simulink model "tests_inverse_shapers"  (R2015b)
settings: Solver=VariableStepAuto  StartTime=0.0  StopTime=10.0  RelTol=1e-3
undefined symbols (not defined in the file): a, alpha, tau
libraries: cstblocks x1
settings Model: Creator=dave  LastModifiedBy=dave

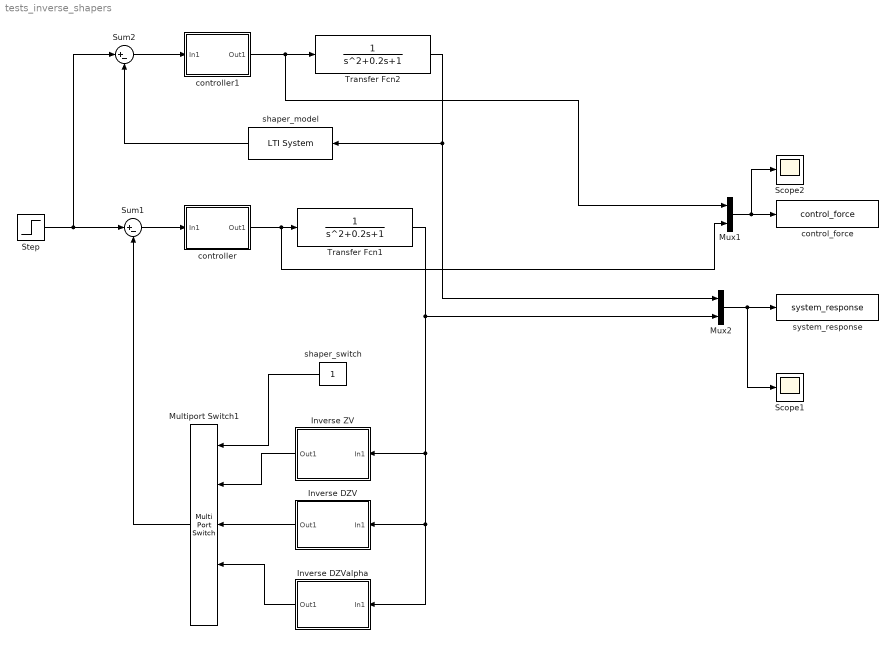
== system tests_inverse_shapers ==
  Inverse DZV : Subsystem
  Inverse DZValpha : Subsystem
  Inverse ZV : Subsystem
  Multiport Switch1 : MultiPortSwitch  Inputs=4
  Mux1 : Mux  Inputs=2
  Mux2 : Mux  Inputs=2
  Scope1 : Scope
  Scope2 : Scope
  Step : Step  SampleTime=0
  Sum1 : Sum  Inputs=|+-
  Sum2 : Sum  Inputs=|+-
  Transfer Fcn1 : TransferFcn  Denominator=[1 0.2 1]
  Transfer Fcn2 : TransferFcn  Denominator=[1 0.2 1]
  control_force : ToWorkspace  VariableName=control_force  SaveFormat=Timeseries  SampleTime=-1
  controller : Subsystem
  controller1 : Subsystem
  shaper_model : cstblocks/LTI System  sys=shaper_model  IC=[]
  shaper_switch : Constant
  system_response : ToWorkspace  VariableName=system_response  SaveFormat=Timeseries  SampleTime=-1
  wires:
  Step/1 -> Sum2/1, Sum1/1
  Sum1/1 -> controller/1(In1)
  controller/1(Out1) -> Mux1/2, Transfer Fcn1/1
  Sum2/1 -> controller1/1(In1)
  controller1/1(Out1) -> Mux1/1, Transfer Fcn2/1
  shaper_model/1 -> Sum2/2
  Mux2/1 -> Scope1/1, system_response/1
  Transfer Fcn2/1 -> Mux2/1, shaper_model/1
  Transfer Fcn1/1 -> Inverse DZValpha/1(In1), Inverse DZV/1(In1), Inverse ZV/1(In1), Mux2/2
  Mux1/1 -> Scope2/1, control_force/1
  Inverse DZValpha/1(Out1) -> Multiport Switch1/4
  Inverse DZV/1(Out1) -> Multiport Switch1/3
  Inverse ZV/1(Out1) -> Multiport Switch1/2
  shaper_switch/1 -> Multiport Switch1/1
  Multiport Switch1/1 -> Sum1/2

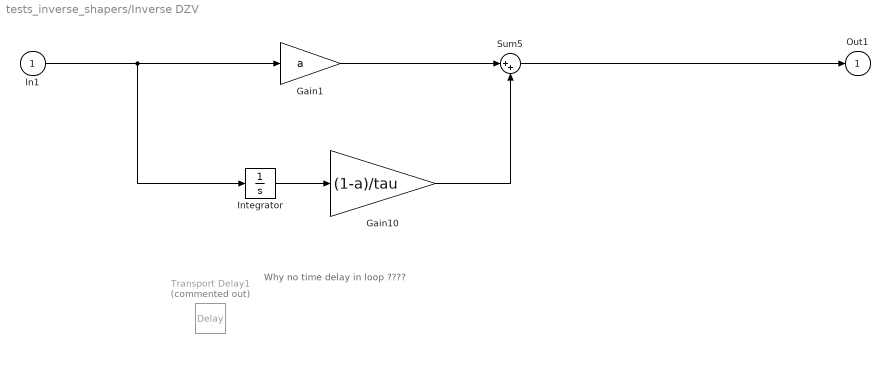
== system tests_inverse_shapers/Inverse DZV ==
  note: Why no time delay in loop ????
  In1 : Inport
  Gain1 : Gain  Gain=a
  Gain10 : Gain  Gain=(1-a)/tau
  Integrator : Integrator  LimitOutput=on  UpperSaturationLimit=tau  LowerSaturationLimit=0
  Sum5 : Sum  Inputs=|++
  Transport Delay1 : TransportDelay  Commented=on  DelayTime=tau
  Out1 : Outport
  wires:
  Sum5/1 -> Out1/1
  Integrator/1 -> Gain10/1
  Gain10/1 -> Sum5/2
  Gain1/1 -> Sum5/1
  In1/1 -> Integrator/1, Gain1/1

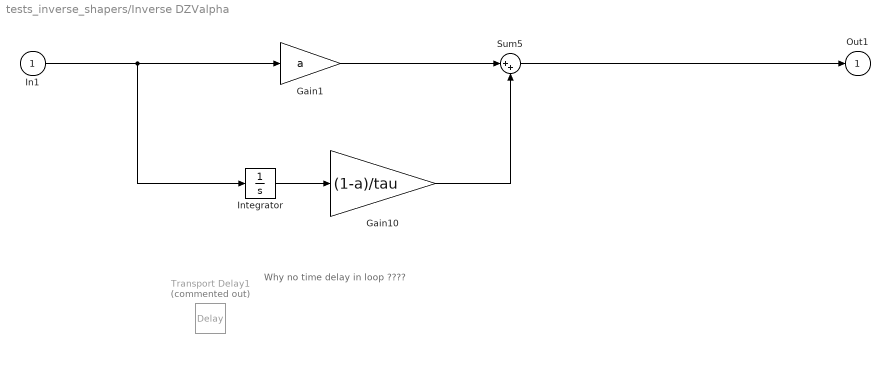
== system tests_inverse_shapers/Inverse DZValpha ==
  note: Why no time delay in loop ????
  In1 : Inport
  Gain1 : Gain  Gain=a
  Gain10 : Gain  Gain=(1-a)/tau
  Integrator : Integrator  LimitOutput=on  UpperSaturationLimit=tau  LowerSaturationLimit=0
  Sum5 : Sum  Inputs=|++
  Transport Delay1 : TransportDelay  Commented=on  DelayTime=tau
  Out1 : Outport
  wires:
  In1/1 -> Gain1/1, Integrator/1
  Gain1/1 -> Sum5/1
  Gain10/1 -> Sum5/2
  Integrator/1 -> Gain10/1
  Sum5/1 -> Out1/1

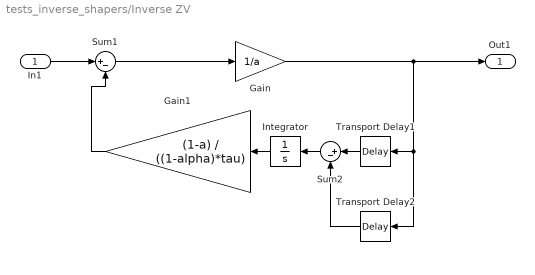
== system tests_inverse_shapers/Inverse ZV ==
  In1 : Inport
  Gain : Gain  Gain=1/a
  Gain1 : Gain  Gain=(1-a) / ((1-alpha)*tau)
  Integrator : Integrator  LimitOutput=on  UpperSaturationLimit=tau  LowerSaturationLimit=0
  Sum1 : Sum  Inputs=|+-
  Sum2 : Sum  Inputs=|+-
  Transport Delay1 : TransportDelay  DelayTime=tau*alpha
  Transport Delay2 : TransportDelay  DelayTime=tau
  Out1 : Outport
  wires:
  Gain/1 -> Transport Delay2/1, Transport Delay1/1, Out1/1
  Gain1/1 -> Sum1/2
  Sum1/1 -> Gain/1
  In1/1 -> Sum1/1
  Integrator/1 -> Gain1/1
  Transport Delay2/1 -> Sum2/2
  Sum2/1 -> Integrator/1
  Transport Delay1/1 -> Sum2/1

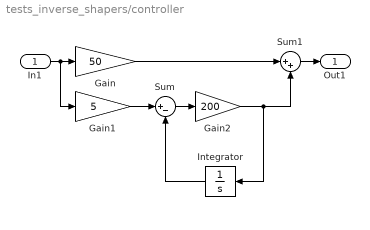
== system tests_inverse_shapers/controller ==
  In1 : Inport
  Gain : Gain  Gain=50
  Gain1 : Gain  Gain=5
  Gain2 : Gain  Gain=200
  Integrator : Integrator
  Sum : Sum  Inputs=|+-
  Sum1 : Sum  Inputs=|++
  Out1 : Outport
  wires:
  Gain/1 -> Sum1/1
  Gain1/1 -> Sum/1
  In1/1 -> Gain1/1, Gain/1
  Sum/1 -> Gain2/1
  Gain2/1 -> Sum1/2, Integrator/1
  Integrator/1 -> Sum/2
  Sum1/1 -> Out1/1

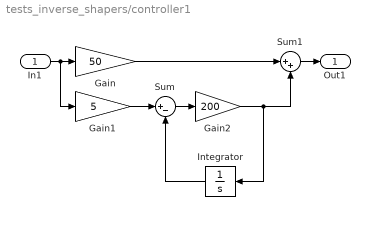
== system tests_inverse_shapers/controller1 ==
  In1 : Inport
  Gain : Gain  Gain=50
  Gain1 : Gain  Gain=5
  Gain2 : Gain  Gain=200
  Integrator : Integrator
  Sum : Sum  Inputs=|+-
  Sum1 : Sum  Inputs=|++
  Out1 : Outport
  wires:
  Sum1/1 -> Out1/1
  Integrator/1 -> Sum/2
  Gain2/1 -> Integrator/1, Sum1/2
  Sum/1 -> Gain2/1
  In1/1 -> Gain/1, Gain1/1
  Gain1/1 -> Sum/1
  Gain/1 -> Sum1/1
